simulink model "step10_observer_3state"  (R2025a)
settings: Solver=ode45  StartTime=0.0  StopTime=20  MaxStep=0.01  RelTol=1e-3
undefined symbols (not defined in the file or in its folder): A, B, F, K, L
libraries: SignalEditorBlockLib x1
settings Model: Creator=O M E N  LastModifiedBy=O M E N

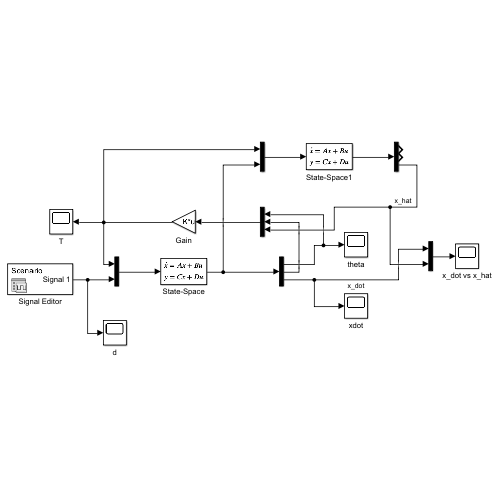
[thumbnail: Simulink's stored preview of the top-level diagram]
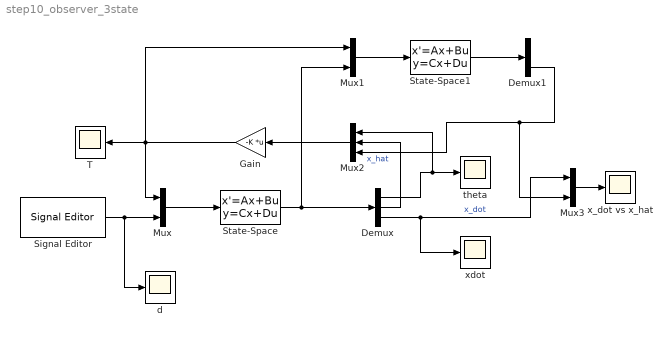
== system step10_observer_3state ==
  Demux : Demux  Outputs=3
  Demux1 : Demux  Outputs=3
  Gain : Gain  Gain=-K  Multiplication=Matrix(K*u)
  Mux : Mux  Inputs=2
  Mux1 : Mux  Inputs=2
  Mux2 : Mux  Inputs=3
  Mux3 : Mux  Inputs=2
  Signal Editor : SignalEditorBlockLib/Signal Editor  FileName=d_trapezoid.mat  ActiveScenario=Scenario  ActiveSignal=Signal 1  IsBus=off  OutputBusObjectStr=Bus: BusObject  SampleTime=0  ZeroCross=off  OutputAfterFinalValue=Setting to zero  Unit=inherit  PreserveSignalName=on  ApplySigPropsToAllScenarios=on  ApplySigPropsToAllSignals=off  SignalPropertySource=Dialog parameters
  State-Space : StateSpace  A=A  B=[B F]  C=eye(3)  D=zeros(3,2)  InitialCondition=[0; 0; 0]
  State-Space1 : StateSpace  A=A - L  B=[B L]  C=eye(3)  D=zeros(3,4)  InitialCondition=[0; 0; 0.05]
  T : Scope
      settings: Title=Control torque T(t)  ActiveDisplayYMinimum=-8.9909489584736342  ActiveDisplayYMaximum=28.2110211862469  YLabel="T  (N·m)"  DataLoggingVariableName=ScopeData2
  d : Scope
      settings: Title=Disturbance d(t)  ActiveDisplayYMinimum=-0.0012499999999999998  ActiveDisplayYMaximum=0.01125  YLabel="d  (m)"  DataLoggingVariableName=ScopeData3
  theta : Scope
      settings: Title=Tilt angle θ(t)  ActiveDisplayYMinimum=-0.011102386767716401  ActiveDisplayYMaximum=0.0015777700092307698  YLabel="θ  (rad)"
  x_dot vs x_hat : Scope
      settings: Title=True vs. estimated speed  ActiveDisplayYMinimum=-0.02618209753717482  ActiveDisplayYMaximum=0.14191539936823308  YLabel="ẋ, ẋ̂  (m/s)"  DataLoggingVariableName=ScopeData4
  xdot : Scope
      settings: Title=Vehicle speed ẋ(t)  ActiveDisplayYMinimum=-0.026182097537174813  ActiveDisplayYMaximum=0.14191539936823305  YLabel="ẋ  (m/s)"
  wires:
  Mux/1 -> State-Space/1
  State-Space/1 -> Mux1/2, Demux/1
  Gain/1 -> Mux1/1, T/1, Mux/1
  Signal Editor/1 -> d/1, Mux/2
  Demux/1 -> Mux2/1, theta/1
  Demux/3 -> Mux3/1, xdot/1  "x_dot"
  Mux1/1 -> State-Space1/1
  State-Space1/1 -> Demux1/1
  Demux/2 -> Mux2/2
  Demux1/3 -> Mux3/2, Mux2/3  "x_hat"
  Mux2/1 -> Gain/1
  Mux3/1 -> x_dot vs x_hat/1
